simulink subsystem "PumpDummyTh"  (R2024b)
settings: Solver=VariableStepAuto  StartTime=0.0  StopTime=10.0  RelTol=1e-3
model mask{pumpMaxCurrent=pump.pumpMaxCurrent, coolant_pipe_D=pump.coolant_pipe_D}
  mask prompts: pumpMaxCurrent "[A] Fixed current draw at full command"; coolant_pipe_D "[m] Coolant pipe diameter"
libraries: fl_lib x4, nesl_utility x2
Description:
  | Minimal pump stub with fixed electrical load. Draws I_fixed * PumpCmd from the LV bus. Coolant passes through with no active pumping. Same port interface as Pump.slx.
settings Model: Creator=jjha  LastModifiedBy=jjha

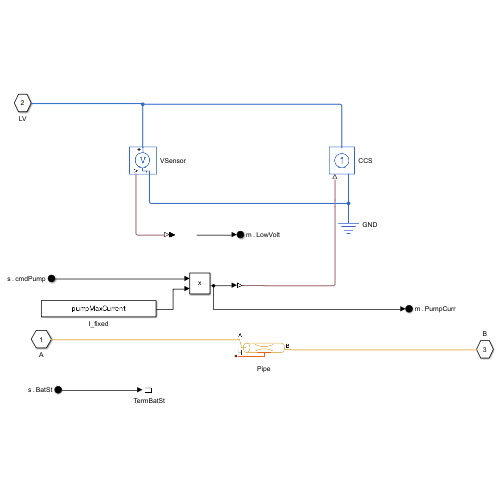
[thumbnail: Simulink's stored preview of the top-level diagram]
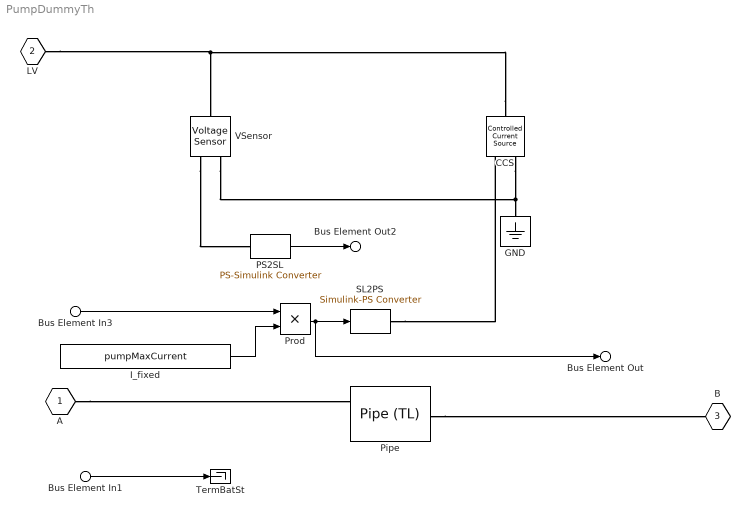
== system PumpDummyTh ==
  Bus Element In1 : Inport  PortName=s  Element=BatSt
  Bus Element In3 : Inport  PortName=s  Element=cmdPump
  CCS : fl_lib/Electrical/Electrical Sources/Controlled Current Source
  GND : fl_lib/Electrical/Electrical Elements/Electrical Reference
  I_fixed : Constant  Value=pumpMaxCurrent
  PS2SL : nesl_utility/PS-Simulink Converter  PhysicalDomain=network_engine_domain  SubClassName=ps_output  LeftPortType=input  RightPortType=output  PseudoPeriodic=off  Frequencies=[]  VectorFormat=inherit  Unit=inherit  AffineConversion=off
  Pipe : fl_lib/Thermal Liquid/Elements/Pipe (TL)  length=5 m  area=0.01 m^2  Dh=0.1128 m  length_add=1 m  roughness=15e-6 m  Re_lam=2000  Re_tur=4000  shape_factor=64  Nu_lam=3.66  dynamic_compressibility=true  inertia=false  p0=0.101325 MPa  T0=293.15 K  mdot0=0 kg/s
  Prod : Product
  SL2PS : nesl_utility/Simulink-PS Converter  PhysicalDomain=network_engine_domain  SubClassName=ps_input  LeftPortType=input  RightPortType=output  PseudoPeriodic=off  Frequencies=[]  NoiseDistribution=none  NoiseParameters=[]  Unit=1  AffineConversion=off  FilteringAndDerivatives=provide  SimscapeFilterOrder=1  InputFilterTimeConstant=0.001  UdotUserProvided=0
  TermBatSt : Terminator
  VSensor : fl_lib/Electrical/Electrical Sensors/Voltage Sensor
  A : PMIOPort  Side=Left
  LV : PMIOPort  Port=2  Side=Left
  B : PMIOPort  Port=3  Side=Right
  Bus Element Out : Outport  PortName=m  Element=PumpCurr
  Bus Element Out2 : Outport  PortName=m  Element=LowVolt
  wires:
  Bus Element In1/1 -> TermBatSt/1
  Bus Element In3/1 -> Prod/1
  I_fixed/1 -> Prod/2
  Prod/1 -> Bus Element Out/1, SL2PS/1
  PS2SL/1 -> Bus Element Out2/1
  connections:
  VSensor/RConn2 -- GND/LConn1 -- CCS/RConn2
  CCS/LConn1 -- LV/RConn1 -- VSensor/LConn1
  VSensor/RConn1 -- PS2SL/LConn1
  SL2PS/RConn1 -- CCS/RConn1
  A/RConn1 -- Pipe/LConn1
  Pipe/RConn1 -- B/RConn1
